simulink model "LV25P"  (R2020b)
settings: Solver=VariableStepAuto  StartTime=0.0  StopTime=1/15  RelTol=1e-3
libraries: fl_lib x14, nesl_utility x6
settings Model: Creator=MrNobody  LastModifiedBy=MrNobody

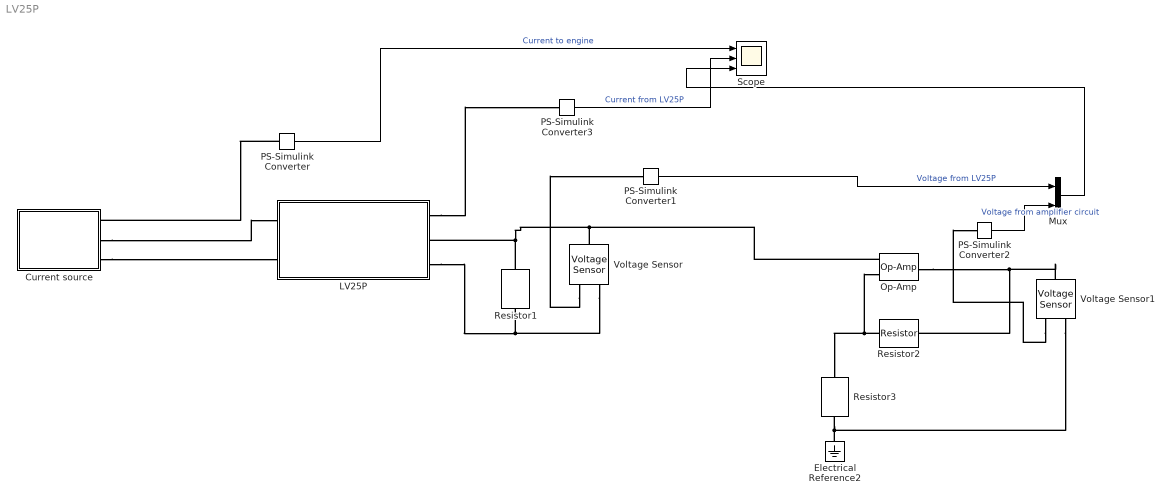
== system LV25P ==
  Current source : Subsystem
  Electrical Reference2 : fl_lib/Electrical/Electrical Elements/Electrical Reference
  LV25P : Subsystem
  Mux : Mux  Inputs=2
  Op-Amp : fl_lib/Electrical/Electrical Elements/Op-Amp  outI_specify=off  outI_priority=None  outI=0 A  outI_nominal_specify=off  outI_nominal_unit=A  outI_nominal_value=1
  PS-Simulink Converter{,1..3} (4 alike) : nesl_utility/PS-Simulink Converter  PhysicalDomain=network_engine_domain  SubClassName=ps_output  LeftPortType=input  RightPortType=output  PseudoPeriodic=off  Frequencies=[]  Unit=inherit  AffineConversion=off
  Resistor1 : fl_lib/Electrical/Electrical Elements/Resistor  R=100 Ohm  i_specify=off  i_priority=None  i=0 A  i_nominal_specify=off  i_nominal_unit=A  i_nominal_value=1  v_specify=off  v_priority=None  v=0 V  v_nominal_specify=off  v_nominal_unit=V  v_nominal_value=1
  Resistor2 : fl_lib/Electrical/Electrical Elements/Resistor  R=30 kOhm  i_specify=off  i_priority=None  i=0 A  i_nominal_specify=off  i_nominal_unit=A  i_nominal_value=1  v_specify=off  v_priority=None  v=0 V  v_nominal_specify=off  v_nominal_unit=V  v_nominal_value=1
  Resistor3 : fl_lib/Electrical/Electrical Elements/Resistor  R=10 kOhm  i_specify=off  i_priority=None  i=0 A  i_nominal_specify=off  i_nominal_unit=A  i_nominal_value=1  v_specify=off  v_priority=None  v=0 V  v_nominal_specify=off  v_nominal_unit=V  v_nominal_value=1
  Scope : Scope  NumInputPorts=3
  Voltage Sensor : fl_lib/Electrical/Electrical Sensors/Voltage Sensor
  Voltage Sensor1 : fl_lib/Electrical/Electrical Sensors/Voltage Sensor
  wires:
  PS-Simulink Converter/1 -> Scope/1  "Current to engine"
  PS-Simulink Converter2/1 -> Mux/2  "Voltage from amplifier circuit"
  PS-Simulink Converter1/1 -> Mux/1  "Voltage from LV25P"
  Mux/1 -> Scope/3
  PS-Simulink Converter3/1 -> Scope/2  "Current from LV25P"
  connections:
  Resistor1/LConn1 -- Op-Amp/LConn1 -- Voltage Sensor/LConn1 -- LV25P/RConn2
  Voltage Sensor/RConn1 -- PS-Simulink Converter1/LConn1
  Electrical Reference2/LConn1 -- Voltage Sensor1/RConn2 -- Resistor3/RConn1
  Resistor2/LConn1 -- Op-Amp/LConn2 -- Resistor3/LConn1
  Op-Amp/RConn1 -- Voltage Sensor1/LConn1 -- Resistor2/RConn1
  Voltage Sensor1/RConn1 -- PS-Simulink Converter2/LConn1
  PS-Simulink Converter/LConn1 -- Current source/RConn1
  Voltage Sensor/RConn2 -- LV25P/RConn3 -- Resistor1/RConn1
  Current source/RConn2 -- LV25P/LConn1
  Current source/RConn3 -- LV25P/LConn2
  LV25P/RConn1 -- PS-Simulink Converter3/LConn1

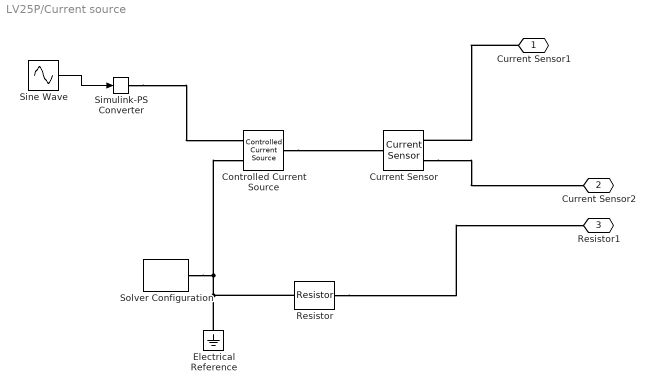
== system LV25P/Current source ==
  Controlled Current Source : fl_lib/Electrical/Electrical Sources/Controlled Current Source
  Current Sensor : fl_lib/Electrical/Electrical Sensors/Current Sensor
  Electrical Reference : fl_lib/Electrical/Electrical Elements/Electrical Reference
  Resistor : fl_lib/Electrical/Electrical Elements/Resistor  R=1 Ohm  i_specify=off  i_priority=None  i=0 A  i_nominal_specify=off  i_nominal_unit=A  i_nominal_value=1  v_specify=off  v_priority=None  v=0 V  v_nominal_specify=off  v_nominal_unit=V  v_nominal_value=1
  Simulink-PS Converter : nesl_utility/Simulink-PS Converter  PhysicalDomain=network_engine_domain  SubClassName=ps_input  LeftPortType=input  RightPortType=output  PseudoPeriodic=off  Frequencies=[]  NoiseDistribution=none  NoiseParameters=[]  Unit=1  AffineConversion=off  FilteringAndDerivatives=provide  SimscapeFilterOrder=1  InputFilterTimeConstant=0.001  UdotUserProvided=0
  Sine Wave : Sin  Amplitude=200  Frequency=200  SampleTime=0
  Solver Configuration : nesl_utility/Solver Configuration  PhysicalDomain=network_engine_domain  SubClassName=solver  LeftPortType=input  RightPortType=generic  Tones=[]  Harmonics=[]  SimulateNoise=off  Profile=off  UseLocalSampling=off  EnableSwitchedLinearOptims=on  FrequencyDomain=off  UseCCode=off  RelTol=0.001  AbsTol=1e-06  MinStep=1e-09  ToWorkspace=off  RevertToSquareIcSolve=off  NumHomotopyIterations=100  PhasorMode=off  PhasorModeNumHarmonics=1  DoDC=off  ResidualTolerance=1e-09  UseLocalSolver=off  LocalSolverChoice=NE_BACKWARD_EULER_ADVANCER  LocalSolverSampleTime=0.001  DoFixedCost=off  MaxNonlinIter=3  MaxModeIter=2  ComputeImpulses=off  ImpulseIterations=2  LinearAlgebra=auto  EquationFormulation=NE_TIME_EF  DelaysMemoryBudget=1024  AutomaticFiltering=on  FilteringTimeConstant=0.001  PartitionStorageMethod=AS_NEEDED  PartitionMemoryBudget=1024  PartitionMethod=ROBUST
  Current Sensor1 : PMIOPort  Side=Right
  Current Sensor2 : PMIOPort  Port=2  Side=Right
  Resistor1 : PMIOPort  Port=3  Side=Right
  wires:
  Sine Wave/1 -> Simulink-PS Converter/1
  connections:
  Electrical Reference/LConn1 -- Resistor/LConn1 -- Solver Configuration/RConn1 -- Controlled Current Source/RConn2
  Resistor/RConn1 -- Resistor1/RConn1
  Simulink-PS Converter/RConn1 -- Controlled Current Source/RConn1
  Current Sensor1/RConn1 -- Current Sensor/RConn1
  Controlled Current Source/LConn1 -- Current Sensor/LConn1
  Current Sensor/RConn2 -- Current Sensor2/RConn1

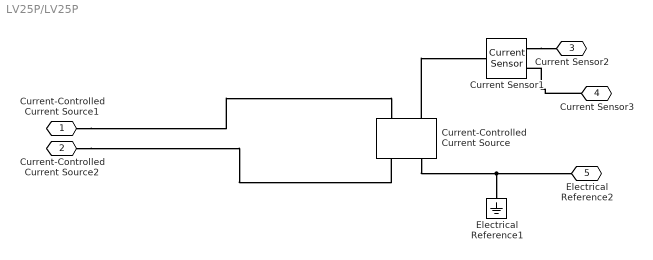
== system LV25P/LV25P ==
  Current Sensor1 : fl_lib/Electrical/Electrical Sensors/Current Sensor
  Current-Controlled Current Source : fl_lib/Electrical/Electrical Sources/Current-Controlled Current Source  K=0.000125  i1_specify=off  i1_priority=None  i1=0 A  i1_nominal_specify=off  i1_nominal_unit=A  i1_nominal_value=1  i2_specify=off  i2_priority=None  i2=0 A  i2_nominal_specify=off  i2_nominal_unit=A  i2_nominal_value=1
      settings: SourceProductBaseCode=SS  InternalSimscapePortConfiguration="{\"Bottom\":[],\"Left\":[{\"id\":\"p1\",\"label\":\"+\",\"type\":\"foundation.electrical.electrical\"},{\"id\":\"head\",\"label\":\"\",\"type\":\"foundation.electrical.electrical\"}],\"Right\":[{\"id\":\"n1\",\"label\":\"-\",\"type\":\"foundation.electrical.electrical\"},{\"id\":\"tail\",\"label\":\"\",\"type\":\"foundation.electrical.electrical\"}],\"Top\":[]}"
  Electrical Reference1 : fl_lib/Electrical/Electrical Elements/Electrical Reference
  Current-Controlled Current Source1 : PMIOPort  Side=Left
  Current-Controlled Current Source2 : PMIOPort  Port=2  Side=Left
  Current Sensor2 : PMIOPort  Port=3  Side=Right
  Current Sensor3 : PMIOPort  Port=4  Side=Right
  Electrical Reference2 : PMIOPort  Port=5  Side=Right
  connections:
  Current-Controlled Current Source/RConn2 -- Electrical Reference2/RConn1 -- Electrical Reference1/LConn1
  Current-Controlled Current Source/LConn2 -- Current Sensor1/LConn1
  Current Sensor3/RConn1 -- Current Sensor1/RConn2
  Current-Controlled Current Source1/RConn1 -- Current-Controlled Current Source/LConn1
  Current-Controlled Current Source2/RConn1 -- Current-Controlled Current Source/RConn1
  Current Sensor1/RConn1 -- Current Sensor2/RConn1
